simulink model "motor_model_3"  (R2018b)
settings: Solver=VariableStepAuto  StartTime=0.0  StopTime=3  RelTol=1e-3
model workspace (MAT data in the model file):
  Ce = 0.14
  Cm = 0.1
  Jsumm = 0.00084
  Kf = 1
  L = 0.001
  R = 0.52
  U = 27
  a = 0
  b = -2.09439510239
  c = 2.09439510239
  poles = 8
libraries: simulink x2
settings Model: Creator=Sainquake  LastModifiedBy=Sainquake

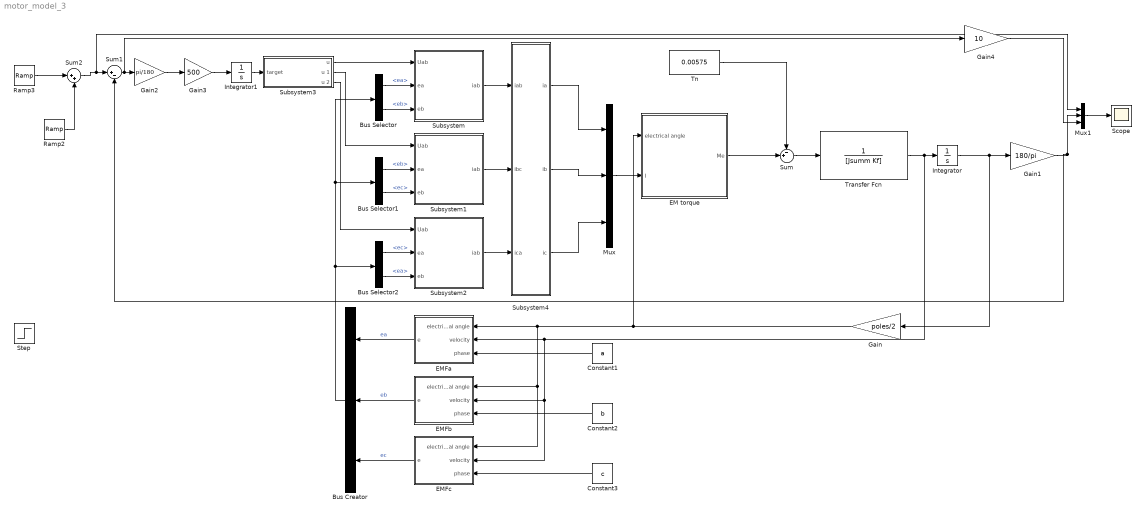
== system motor_model_3 ==
  Bus Creator : BusCreator  Inputs=3
  Bus Selector : BusSelector  OutputSignals=ea,eb
  Bus Selector1 : BusSelector  OutputSignals=eb,ec
  Bus Selector2 : BusSelector  OutputSignals=ec,ea
  Constant1 : Constant  Value=a
  Constant2 : Constant  Value=b
  Constant3 : Constant  Value=c
  EM torque : Subsystem
  EMFa : Subsystem
  EMFb : Subsystem
  EMFc : Subsystem
  Gain : Gain  Gain=poles/2
  Gain1 : Gain  Gain=180/pi
  Gain2 : Gain  Gain=pi/180
  Gain3 : Gain  Gain=500
  Gain4 : Gain  Gain=10
  Integrator : Integrator
  Integrator1 : Integrator
  Mux : Mux  Inputs=3
  Mux1 : Mux  Inputs=3
  Ramp2 : simulink/Sources/Ramp  slope=-90/0.6  start=2  InitialOutput=0
  Ramp3 : simulink/Sources/Ramp  slope=90/0.6  start=1  InitialOutput=0
  Scope : Scope
  Step : Step  After=10  SampleTime=0
  Subsystem : Subsystem
  Subsystem1 : Subsystem
  Subsystem2 : Subsystem
  Subsystem3 : Subsystem
  Subsystem4 : Subsystem
  Sum : Sum  Inputs=-+|
  Sum1 : Sum  Inputs=|+-
  Sum2 : Sum  Inputs=|++
  "Tn " : Constant  Value=0.00575
  Transfer Fcn : TransferFcn  Denominator=[Jsumm Kf]
  wires:
  Subsystem4/3(ic) -> Mux/3
  Subsystem4/2(ib) -> Mux/2
  Mux/1 -> EM torque/2(I)
  EM torque/1(Me) -> Sum/2
  Sum/1 -> Transfer Fcn/1
  Transfer Fcn/1 -> EMFc/2(velocity), EMFb/2(velocity), EMFa/2(velocity), Integrator/1
  Integrator/1 -> Gain1/1, Gain/1
  Gain/1 -> EM torque/1(electrical angle), EMFc/1(electrical angle), EMFb/1(electrical angle), EMFa/1(electrical angle)
  Mux1/1 -> Scope/1
  Gain1/1 -> Sum1/2, Mux1/2
  Sum1/1 -> Gain4/1, Gain2/1
  Ramp3/1 -> Sum2/1
  Constant1/1 -> EMFa/3(phase)
  Constant2/1 -> EMFb/3(phase)
  Constant3/1 -> EMFc/3(phase)
  EMFa/1(e) -> Bus Creator/1  "ea"
  EMFb/1(e) -> Bus Creator/2  "eb"
  EMFc/1(e) -> Bus Creator/3  "ec"
  Bus Creator/1 -> Bus Selector2/1, Bus Selector1/1, Bus Selector/1
  Bus Selector/1 -> Subsystem/2("ea ")  "<ea>"
  Bus Selector/2 -> Subsystem/3(eb)  "<eb>"
  Bus Selector1/1 -> Subsystem1/2("ea ")  "<eb>"
  Bus Selector1/2 -> Subsystem1/3(eb)  "<ec>"
  Bus Selector2/1 -> Subsystem2/2("ea ")  "<ec>"
  Bus Selector2/2 -> Subsystem2/3(eb)  "<ea>"
  Subsystem/1(iab) -> Subsystem4/1(iab)
  Subsystem1/1(iab) -> Subsystem4/2("ibc ")
  Subsystem2/1(iab) -> Subsystem4/3(ica)
  Subsystem4/1(ia) -> Mux/1
  Sum2/1 -> Mux1/1, Sum1/1
  Gain2/1 -> Gain3/1
  Subsystem3/1("u ") -> Subsystem/1(Uab)
  Subsystem3/2(u 1) -> Subsystem1/1(Uab)
  Subsystem3/3(u 2) -> Subsystem2/1(Uab)
  Ramp2/1 -> Sum2/2
  Integrator1/1 -> Subsystem3/1(target)
  Gain3/1 -> Integrator1/1
  Gain4/1 -> Mux1/3
  "Tn "/1 -> Sum/1

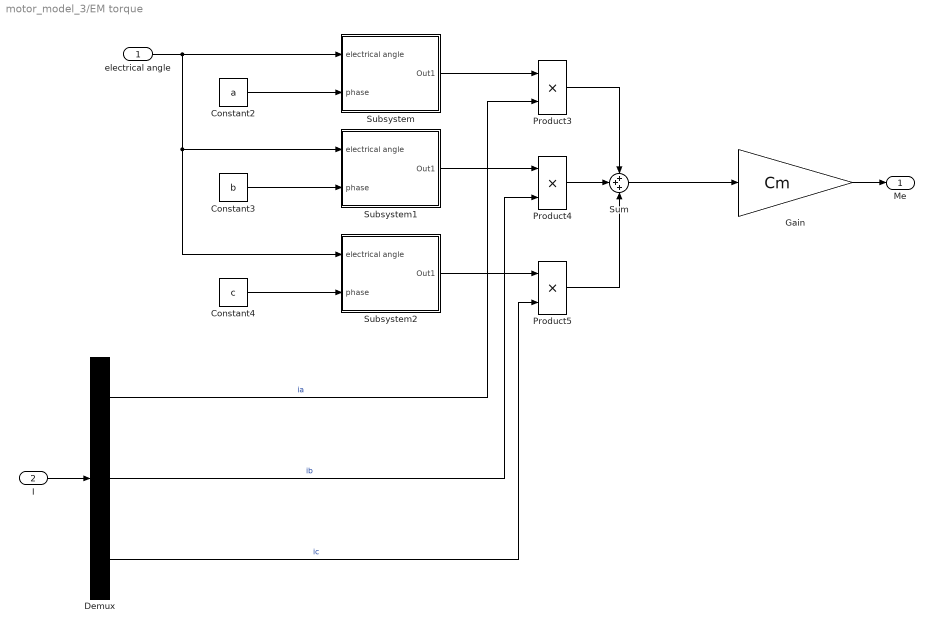
== system motor_model_3/EM torque ==
  electrical angle : Inport
  I : Inport  Port=2
  Constant2 : Constant  Value=a
  Constant3 : Constant  Value=b
  Constant4 : Constant  Value=c
  Demux : Demux  Outputs=3
  Gain : Gain  Gain=Cm
  Product3 : Product
  Product4 : Product
  Product5 : Product
  Subsystem : Subsystem
  Subsystem1 : Subsystem
  Subsystem2 : Subsystem
  Sum : Sum  Inputs=+++
  Me : Outport
  wires:
  Sum/1 -> Gain/1
  Gain/1 -> Me/1
  I/1 -> Demux/1
  Constant2/1 -> Subsystem/2(phase)
  electrical angle/1 -> Subsystem2/1(electrical angle), Subsystem1/1(electrical angle), Subsystem/1(electrical angle)
  Constant3/1 -> Subsystem1/2(phase)
  Constant4/1 -> Subsystem2/2(phase)
  Demux/1 -> Product3/2  "ia"
  Subsystem/1(Out1) -> Product3/1
  Demux/2 -> Product4/2  "ib"
  Demux/3 -> Product5/2  "ic"
  Subsystem1/1(Out1) -> Product4/1
  Subsystem2/1(Out1) -> Product5/1
  Product4/1 -> Sum/2
  Product3/1 -> Sum/1
  Product5/1 -> Sum/3

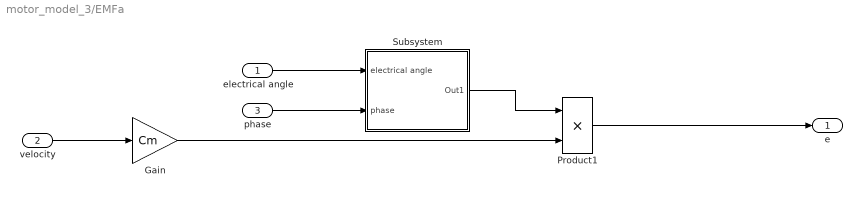
== system motor_model_3/EMFa ==
  electrical angle : Inport
  velocity : Inport  Port=2
  phase : Inport  Port=3
  Gain : Gain  Gain=Cm
  Product1 : Product
  Subsystem : Subsystem
  e : Outport
  wires:
  Gain/1 -> Product1/2
  Product1/1 -> e/1
  velocity/1 -> Gain/1
  phase/1 -> Subsystem/2(phase)
  electrical angle/1 -> Subsystem/1(electrical angle)
  Subsystem/1(Out1) -> Product1/1

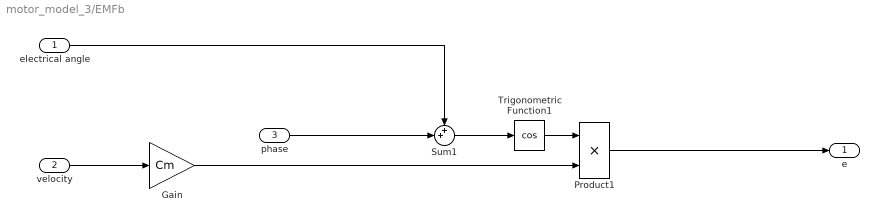
== system motor_model_3/EMFb ==
  electrical angle : Inport
  velocity : Inport  Port=2
  phase : Inport  Port=3
  Gain : Gain  Gain=Cm
  Product1 : Product
  Sum1 : Sum  Inputs=++|
  Trigonometric Function1 : Trigonometry  Operator=cos
  e : Outport
  wires:
  Trigonometric Function1/1 -> Product1/1
  Gain/1 -> Product1/2
  Sum1/1 -> Trigonometric Function1/1
  phase/1 -> Sum1/2
  electrical angle/1 -> Sum1/1
  Product1/1 -> e/1
  velocity/1 -> Gain/1

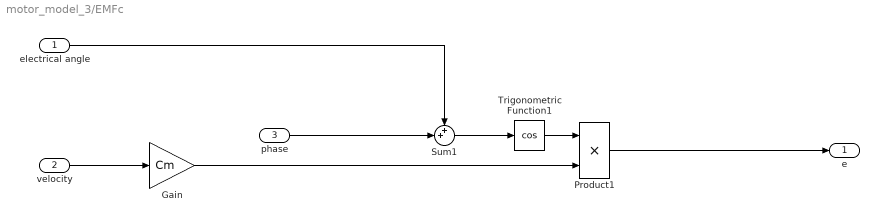
== system motor_model_3/EMFc ==
  electrical angle : Inport
  velocity : Inport  Port=2
  phase : Inport  Port=3
  Gain : Gain  Gain=Cm
  Product1 : Product
  Sum1 : Sum  Inputs=++|
  Trigonometric Function1 : Trigonometry  Operator=cos
  e : Outport
  wires:
  Trigonometric Function1/1 -> Product1/1
  Gain/1 -> Product1/2
  Sum1/1 -> Trigonometric Function1/1
  phase/1 -> Sum1/2
  electrical angle/1 -> Sum1/1
  Product1/1 -> e/1
  velocity/1 -> Gain/1

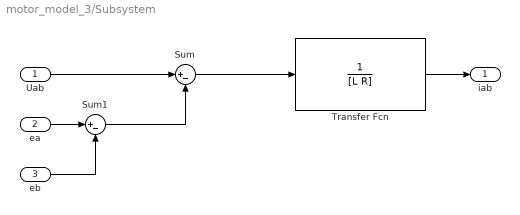
== system motor_model_3/Subsystem ==
  Uab : Inport
  "ea " : Inport  Port=2
  eb : Inport  Port=3
  Sum : Sum  Inputs=|+-
  Sum1 : Sum  Inputs=|+-
  Transfer Fcn : TransferFcn  Denominator=[L R]
  iab : Outport
  wires:
  Uab/1 -> Sum/1
  Transfer Fcn/1 -> iab/1
  Sum/1 -> Transfer Fcn/1
  "ea "/1 -> Sum1/1
  eb/1 -> Sum1/2
  Sum1/1 -> Sum/2

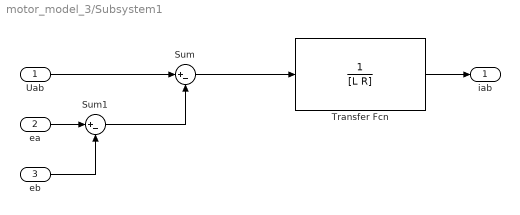
== system motor_model_3/Subsystem1 ==
  Uab : Inport
  "ea " : Inport  Port=2
  eb : Inport  Port=3
  Sum : Sum  Inputs=|+-
  Sum1 : Sum  Inputs=|+-
  Transfer Fcn : TransferFcn  Denominator=[L R]
  iab : Outport
  wires:
  Uab/1 -> Sum/1
  Transfer Fcn/1 -> iab/1
  Sum/1 -> Transfer Fcn/1
  "ea "/1 -> Sum1/1
  eb/1 -> Sum1/2
  Sum1/1 -> Sum/2

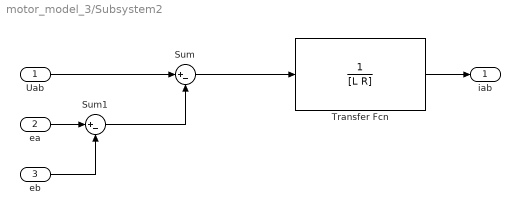
== system motor_model_3/Subsystem2 ==
  Uab : Inport
  "ea " : Inport  Port=2
  eb : Inport  Port=3
  Sum : Sum  Inputs=|+-
  Sum1 : Sum  Inputs=|+-
  Transfer Fcn : TransferFcn  Denominator=[L R]
  iab : Outport
  wires:
  Uab/1 -> Sum/1
  Transfer Fcn/1 -> iab/1
  Sum/1 -> Transfer Fcn/1
  "ea "/1 -> Sum1/1
  eb/1 -> Sum1/2
  Sum1/1 -> Sum/2

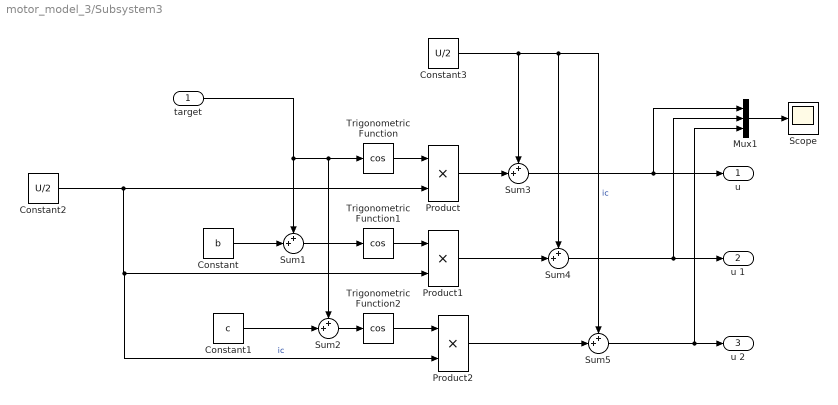
== system motor_model_3/Subsystem3 ==
  target : Inport
  Constant : Constant  Value=b
  Constant1 : Constant  Value=c
  Constant2 : Constant  Value=U/2
  Constant3 : Constant  Value=U/2
  Mux1 : Mux  Inputs=3
  Product : Product
  Product1 : Product
  Product2 : Product
  Scope : Scope
  Sum{1..5} (5 alike) : Sum  Inputs=++|
  Trigonometric Function : Trigonometry  Operator=cos
  Trigonometric Function1 : Trigonometry  Operator=cos
  Trigonometric Function2 : Trigonometry  Operator=cos
  "u " : Outport
  u 1 : Outport  Port=2
  u 2 : Outport  Port=3
  wires:
  Sum3/1 -> Mux1/1, "u "/1
  target/1 -> Sum2/1, Trigonometric Function/1, Sum1/1
  Trigonometric Function2/1 -> Product2/1
  Sum2/1 -> Trigonometric Function2/1
  Trigonometric Function1/1 -> Product1/1
  Constant2/1 -> Product/2, Product2/2, Product1/2  "ic"
  Constant1/1 -> Sum2/2
  Sum1/1 -> Trigonometric Function1/1
  Constant/1 -> Sum1/2
  Trigonometric Function/1 -> Product/1
  Constant3/1 -> Sum5/1, Sum4/1, Sum3/1  "ic"
  Product/1 -> Sum3/2
  Product1/1 -> Sum4/2
  Product2/1 -> Sum5/2
  Sum5/1 -> Mux1/3, u 2/1
  Sum4/1 -> Mux1/2, u 1/1
  Mux1/1 -> Scope/1

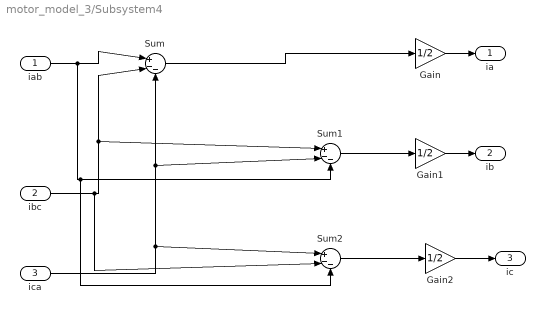
== system motor_model_3/Subsystem4 ==
  iab : Inport
  "ibc " : Inport  Port=2
  ica : Inport  Port=3
  Gain : Gain  Gain=1/2
  Gain1 : Gain  Gain=1/2
  Gain2 : Gain  Gain=1/2
  Sum : Sum  Inputs=|+--
  Sum1 : Sum  Inputs=|+--
  Sum2 : Sum  Inputs=|+--
  ia : Outport
  ib : Outport  Port=2
  ic : Outport  Port=3
  wires:
  Gain/1 -> ia/1
  Gain1/1 -> ib/1
  Gain2/1 -> ic/1
  iab/1 -> Sum2/3, Sum1/3, Sum/1
  "ibc "/1 -> Sum2/2, Sum1/1, Sum/2
  ica/1 -> Sum2/1, Sum1/2, Sum/3
  Sum/1 -> Gain/1
  Sum1/1 -> Gain1/1
  Sum2/1 -> Gain2/1

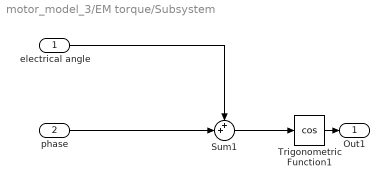
== system motor_model_3/EM torque/Subsystem ==
  electrical angle : Inport
  phase : Inport  Port=2
  Sum1 : Sum  Inputs=++|
  Trigonometric Function1 : Trigonometry  Operator=cos
  Out1 : Outport
  wires:
  electrical angle/1 -> Sum1/1
  Sum1/1 -> Trigonometric Function1/1
  phase/1 -> Sum1/2
  Trigonometric Function1/1 -> Out1/1

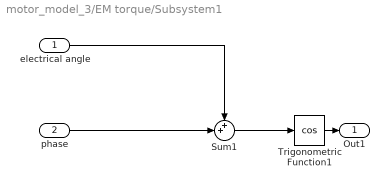
== system motor_model_3/EM torque/Subsystem1 ==
  electrical angle : Inport
  phase : Inport  Port=2
  Sum1 : Sum  Inputs=++|
  Trigonometric Function1 : Trigonometry  Operator=cos
  Out1 : Outport
  wires:
  electrical angle/1 -> Sum1/1
  Sum1/1 -> Trigonometric Function1/1
  phase/1 -> Sum1/2
  Trigonometric Function1/1 -> Out1/1

== system motor_model_3/EM torque/Subsystem2 ==
  electrical angle : Inport
  phase : Inport  Port=2
  Sum1 : Sum  Inputs=++|
  Trigonometric Function1 : Trigonometry  Operator=cos
  Out1 : Outport
  wires:
  electrical angle/1 -> Sum1/1
  Sum1/1 -> Trigonometric Function1/1
  phase/1 -> Sum1/2
  Trigonometric Function1/1 -> Out1/1

== system motor_model_3/EMFa/Subsystem ==
  electrical angle : Inport
  phase : Inport  Port=2
  Sum1 : Sum  Inputs=++|
  Trigonometric Function1 : Trigonometry  Operator=cos
  Out1 : Outport
  wires:
  electrical angle/1 -> Sum1/1
  Sum1/1 -> Trigonometric Function1/1
  phase/1 -> Sum1/2
  Trigonometric Function1/1 -> Out1/1
